simulink model "Part1_3_c"  (R2019a)
settings: Solver=VariableStepAuto  StartTime=0.0  StopTime=24  RelTol=1e-3
libraries: robotalgslib x1, simulink x1
settings Model: Creator=Admin  LastModifiedBy=admin
settings DebuggingCC: UnderSpecifiedDimensionMsg=warning

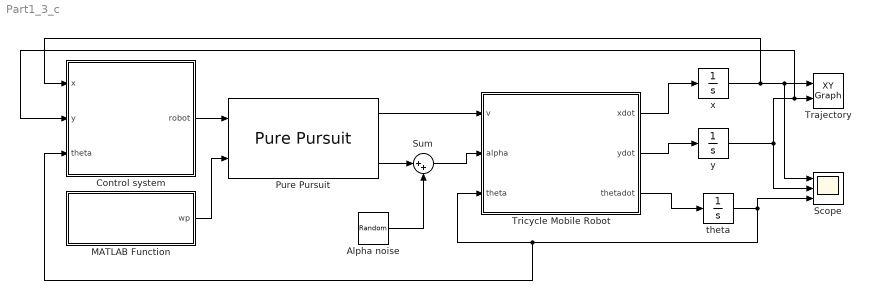
== system Part1_3_c ==
  Alpha noise : UniformRandomNumber  Minimum=0  Maximum=5*pi/180  SampleTime=0.1
  Control system : MATLAB Function  TreatAsAtomicUnit=on
  MATLAB Function : MATLAB Function  TreatAsAtomicUnit=on
  Pure Pursuit : robotalgslib/Pure Pursuit  DesiredLinearVelocity=1.95  MaxAngularVelocity=0.3  LookaheadDistance=1  TargetDirPort=on  SimulateUsing=Code generation
      settings: SourceProductName=Navigation Toolbox  SourceProductBaseCode=NV
  Scope : Scope  NumInputPorts=3
  Sum : Sum  Inputs=|++
  Trajectory : simulink/Sinks/XY Graph  xmin=-1  xmax=25  ymin=-10  ymax=6  st=-1
  Tricycle Mobile Robot : MATLAB Function  TreatAsAtomicUnit=on
  theta : Integrator
  x : Integrator
  y : Integrator
  wires:
  y/1 -> Control system/2(y), Trajectory/2, Scope/2
  Tricycle Mobile Robot/1(xdot) -> x/1
  Tricycle Mobile Robot/3(thetadot) -> theta/1
  Tricycle Mobile Robot/2(ydot) -> y/1
  x/1 -> Control system/1(x), Scope/1, Trajectory/1
  theta/1 -> Control system/3(theta), Tricycle Mobile Robot/3(theta), Scope/3
  Control system/1(robot) -> Pure Pursuit/1
  Pure Pursuit/1 -> Tricycle Mobile Robot/1(v)
  MATLAB Function/1(wp) -> Pure Pursuit/2
  Pure Pursuit/3 -> Sum/1
  Sum/1 -> Tricycle Mobile Robot/2(alpha)
  Alpha noise/1 -> Sum/2

== matlab function Part1_3_c/Control system ==
  data: x input; robot output; y input; theta input
function robot  = position(x,y,theta)
    robot = [x y theta];
end

== matlab function Part1_3_c/Tricycle Mobile Robot ==
  data: v input; alpha input; xdot output; theta input; ydot output; thetadot output
function [xdot,ydot,thetadot] = Tricycle_type_2(v,alpha,theta)
    d = sqrt(3.1);
    xdot = v*cos(theta);
    ydot = v*sin(theta);
    thetadot = v*tan(alpha)/d; 
end

== matlab function Part1_3_c/MATLAB Function ==
  data: wp output
function wp  = waypoint_PurePursuit()
    wp = [4 0; 8 0; 12 0; 16 0; 20 0; 22 -2; 20 -4; 16 -4; 12 -4; 8 -4; 4 -4;0 -4]
end
